simulink model "schema"  (R2017b)
settings: Solver=VariableStepDiscrete  StartTime=0.0  StopTime=10.0  RelTol=1e-3
libraries: fillib x1
settings Model: Creator=test  LastModifiedBy=test

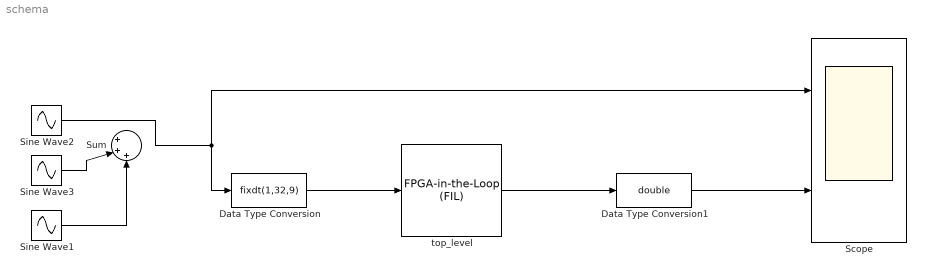
== system schema ==
  Data Type Conversion : DataTypeConversion  OutDataTypeStr=fixdt(1,32,9)
  Data Type Conversion1 : DataTypeConversion  OutDataTypeStr=double
  Scope : Scope  NumInputPorts=2
  Sine Wave1 : Sin  Amplitude=20  Frequency=10  Phase=3.14159  SampleTime=5e-4
  Sine Wave2 : Sin  Amplitude=20  Frequency=20  SampleTime=5e-4
  Sine Wave3 : Sin  Amplitude=20  Frequency=100  SampleTime=5e-4
  Sum : Sum  Inputs=|+++
  top_level : fillib/FPGA-in-the-Loop (FIL)  ForceInterfaceUpdate=0.90579
  wires:
  top_level/1 -> Data Type Conversion1/1
  Sine Wave2/1 -> Scope/1, Data Type Conversion/1
  Data Type Conversion1/1 -> Scope/2
  Data Type Conversion/1 -> top_level/1
  Sine Wave3/1 -> Sum/2
  Sine Wave1/1 -> Sum/3
